simulink library "unit_testing"  (R2012b)
settings: Solver=ode45  StartTime=0.0  StopTime=10.0  RelTol=1e-3
libraries: xbsIndex_r4 x28
settings Model: Creator=ayoung  LastModifiedBy=ayoung

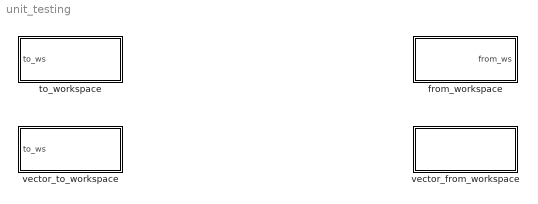
== system unit_testing ==
  from_workspace : Subsystem  mask(from_workspace){n_bits=1, bin_pt=0, arith_type=2, var_name=my_var}
      mask prompts: n_bits "Number of bits"; bin_pt "Binary point"; arith_type "Arithmetic type (ufix=0, fix=1, bool=2)"; var_name "Variable name"
      mask init:
      | blk = from_workspace_init(gcb,...
      |     'n_bits', n_bits,...
      |     'bin_pt',bin_pt,...
      |     'arith_type',arith_type,...
      |     'var_name',var_name);
      mask Display:
      | color('white');
      | text(0.5,0.5,get_param(gcb,'var_name'),'HorizontalAlignment','center');
  to_workspace : Subsystem  mask{var_name=my_var}
      mask prompts: var_name "Variable name"
      mask init:
      | var_inst = [gcb '/mvar'];
      | v = get_param(gcb,'var_name');
      | set_param(var_inst,'VariableName',v);
      mask Display:
      | color('white');
      | text(0.5,0.5,get_param(gcb,'var_name'),'HorizontalAlignment','center');
  vector_from_workspace : Subsystem  mask(vector_from_workspace){n_in=0, n_bits=0, bin_pt=0, arith_type=0, var_pfx=x}
      mask prompts: n_in "Number of inputs"; n_bits "Input width"; bin_pt "Binary point position"; arith_type "Arithmetic type (ufix=0, fix=1, bool=2)"; var_pfx "Variable name prefix"
      mask init:
      | blk = vector_from_workspace_init(gcb,...
      |     'n_in',n_in,...
      |     'n_bits',n_bits,...
      |     'bin_pt',bin_pt,...
      |     'arith_type',arith_type,...
      |     'var_pfx',var_pfx);
      mask Display:
      | color('white');
      | var_pfx = get_param(gcb,'var_pfx');
      | n_1 = 1;
      | n_N = str2num(get_param(gcb,'n_in'));
      | text(0.5,0.5,sprintf('%s_[%d..%d]',var_pfx,n_1,n_N),'HorizontalAlignment','center');
  vector_to_workspace : Subsystem  mask{n_out=8, n_bits=8, bin_pt=7, arith_type=1, var_pfx=x}
      mask prompts: n_out "Number of outputs"; n_bits "Output width"; bin_pt "Binary point position"; arith_type "Arithmetic type (ufix=0, fix=1, bool=2)"; var_pfx "Variable name prefix"
      mask init:
      | bus_inst = [gcb '/bus_expand'];
      | n_out = get_param(gcb,'n_out');
      | n_bits = get_param(gcb,'n_bits');
      | bin_pt = get_param(gcb,'bin_pt');
      | arith_type = get_param(gcb,'arith_type');
      | var_pfx = get_param(gcb,'var_pfx');
      | set_param(bus_inst,'outputNum',n_out);
      | set_param(bus_inst,'outputWidth',n_bits);
      | set_param(bus_inst,'outputBinaryPt',bin_pt);
      | set_param(bus_inst,'outputArithmeticType',arith_type);
      | set_param(bus_inst,'variablePrefix',var_pfx);
      mask Display:
      | color('white');
      | var_pfx = get_param(gcb,'var_pfx');
      | n_1 = 1;
      | n_N = str2num(get_param(gcb,'n_out'));
      | text(0.5,0.5,sprintf('%s_[%d..%d]',var_pfx,n_1,n_N),'HorizontalAlignment','center');

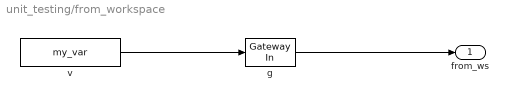
== system unit_testing/from_workspace ==
  g : xbsIndex_r4/Gateway In  gui_display_data_type=Fixed-point  arith_type=Boolean  n_bits=1  bin_pt=0  preci_type=Single  exp_width=8  frac_width=24  quantization="Round  (unbiased: +/- Inf)"  overflow=Saturate  period=1  dbl_ovrd=off  timing_constraint=None  locs_specified=off  LOCs={}  UseAsADC=off  ADCChannel='1'  inherit_from_input=off  hdl_port=on  block_type=gatewayin
  v : FromWorkspace  VariableName=my_var  SampleTime=0
  from_ws : Outport
  wires:
  v/1 -> g/1
  g/1 -> from_ws/1

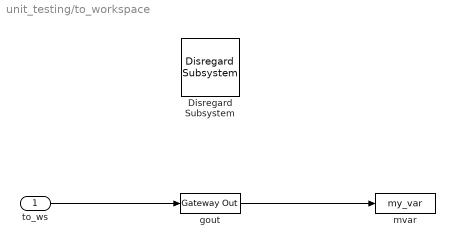
== system unit_testing/to_workspace ==
  to_ws : Inport
  Disregard Subsystem : xbsIndex_r4/Disregard Subsystem  Tag=discardX  block_type=disregard
  gout : xbsIndex_r4/Gateway Out  inherit_from_input=off  hdl_port=on  timing_constraint=None  locs_specified=off  LOCs={}  UseAsDAC=off  DACChannel='1'  block_type=gatewayout
  mvar : ToWorkspace  VariableName=my_var  SampleTime=-1  SaveFormat=Structure With Time
  wires:
  to_ws/1 -> gout/1
  gout/1 -> mvar/1

== system unit_testing/vector_from_workspace ==

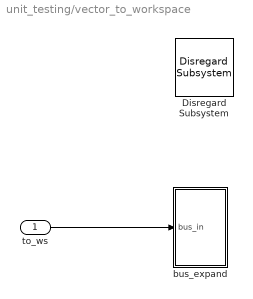
== system unit_testing/vector_to_workspace ==
  to_ws : Inport
  Disregard Subsystem : xbsIndex_r4/Disregard Subsystem  Tag=discardX  block_type=disregard
  bus_expand : Subsystem  AncestorBlock=casper_library_flow_control/bus_expand  mask(bus_expand){mode=divisions of equal size, outputNum=8, outputWidth=8, outputBinaryPt=7, outputArithmeticType=1, show_format=off, outputToWorkspace=on, variablePrefix=x, outputToModelAsWell=off}
      mask prompts: outputNum "Number of outputs:"; outputWidth "Output width:"; outputBinaryPt "Output binary point position:"; outputArithmeticType "Output arithmetic type (ufix=0, fix=1, bool=2):"; show_format "Print format string?"; outputToWorkspace "Output to workspace?"; variablePrefix "Variable name prefix:"; outputToModelAsWell "Output to model as well?"
      mask help:
      | Expands a 'bus' made using a bus_create or Xilinx
      | concat block.
      | The input will be divided into the specified number
      | of outputs with the specified arithmetic types.
      | Divisions are made from most significant bit.
      mask init:
      | bus_expand_init(gcb,...
      |     'mode', mode, ...
      |     'outputNum', outputNum, ...
      |     'outputWidth', outputWidth, ...
      |     'outputBinaryPt', outputBinaryPt, ...
      |     'outputArithmeticType', outputArithmeticType, ...
      |     'show_format', show_format, ...
      |     'outputToWorkspace', outputToWorkspace, ...
      |     'variablePrefix', variablePrefix, ...
      |     'outputToModelAsWell', outputToModelAsWell);
      settings: AttributesFormatString=8 outputs, x_?
      mask TypeOptions mode: divisions of equal size | divisions of arbitrary size
      mask Callback mode: bus_expand_callback();
      mask Callback outputWidth: bus_expand_callback();
      mask Callback outputToWorkspace: bus_expand_callback();
  wires:
  to_ws/1 -> bus_expand/1(bus_in)

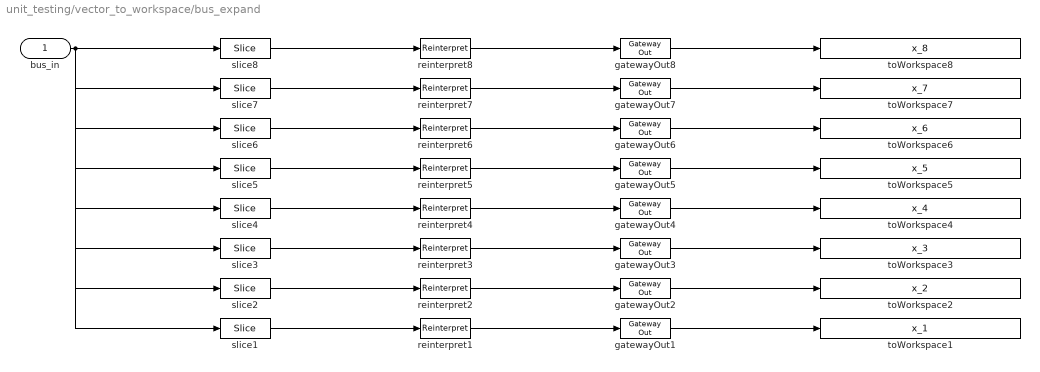
== system unit_testing/vector_to_workspace/bus_expand ==
  bus_in : Inport
  gatewayOut{1..8} (8 alike) : xbsIndex_r4/Gateway Out  inherit_from_input=off  hdl_port=off  timing_constraint=None  locs_specified=off  LOCs={}  UseAsDAC=off  DACChannel='1'  block_type=gatewayout
  reinterpret{1..8} (8 alike) : xbsIndex_r4/Reinterpret  force_arith_type=on  arith_type="Signed  (2's comp)"  force_bin_pt=on  bin_pt=7  block_type=reinterpret
  slice1 : xbsIndex_r4/Slice  nbits=8  boolean_output=off  mode=Upper Bit Location + Width  bit1=-56  base1=MSB of Input  bit0=0  base0=LSB of Input  dbl_ovrd=off  block_type=slice
  slice2 : xbsIndex_r4/Slice  nbits=8  boolean_output=off  mode=Upper Bit Location + Width  bit1=-48  base1=MSB of Input  bit0=0  base0=LSB of Input  dbl_ovrd=off  block_type=slice
  slice3 : xbsIndex_r4/Slice  nbits=8  boolean_output=off  mode=Upper Bit Location + Width  bit1=-40  base1=MSB of Input  bit0=0  base0=LSB of Input  dbl_ovrd=off  block_type=slice
  slice4 : xbsIndex_r4/Slice  nbits=8  boolean_output=off  mode=Upper Bit Location + Width  bit1=-32  base1=MSB of Input  bit0=0  base0=LSB of Input  dbl_ovrd=off  block_type=slice
  slice5 : xbsIndex_r4/Slice  nbits=8  boolean_output=off  mode=Upper Bit Location + Width  bit1=-24  base1=MSB of Input  bit0=0  base0=LSB of Input  dbl_ovrd=off  block_type=slice
  slice6 : xbsIndex_r4/Slice  nbits=8  boolean_output=off  mode=Upper Bit Location + Width  bit1=-16  base1=MSB of Input  bit0=0  base0=LSB of Input  dbl_ovrd=off  block_type=slice
  slice7 : xbsIndex_r4/Slice  nbits=8  boolean_output=off  mode=Upper Bit Location + Width  bit1=-8  base1=MSB of Input  bit0=0  base0=LSB of Input  dbl_ovrd=off  block_type=slice
  slice8 : xbsIndex_r4/Slice  nbits=8  boolean_output=off  mode=Upper Bit Location + Width  bit1=0  base1=MSB of Input  bit0=0  base0=LSB of Input  dbl_ovrd=off  block_type=slice
  toWorkspace1 : ToWorkspace  VariableName=x_1  SampleTime=-1  SaveFormat=Structure With Time
  toWorkspace2 : ToWorkspace  VariableName=x_2  SampleTime=-1  SaveFormat=Structure With Time
  toWorkspace3 : ToWorkspace  VariableName=x_3  SampleTime=-1  SaveFormat=Structure With Time
  toWorkspace4 : ToWorkspace  VariableName=x_4  SampleTime=-1  SaveFormat=Structure With Time
  toWorkspace5 : ToWorkspace  VariableName=x_5  SampleTime=-1  SaveFormat=Structure With Time
  toWorkspace6 : ToWorkspace  VariableName=x_6  SampleTime=-1  SaveFormat=Structure With Time
  toWorkspace7 : ToWorkspace  VariableName=x_7  SampleTime=-1  SaveFormat=Structure With Time
  toWorkspace8 : ToWorkspace  VariableName=x_8  SampleTime=-1  SaveFormat=Structure With Time
  wires:
  bus_in/1 -> slice8/1, slice7/1, slice6/1, slice5/1, slice4/1, slice3/1, slice2/1, slice1/1
  slice8/1 -> reinterpret8/1
  reinterpret8/1 -> gatewayOut8/1
  gatewayOut8/1 -> toWorkspace8/1
  slice7/1 -> reinterpret7/1
  reinterpret7/1 -> gatewayOut7/1
  gatewayOut7/1 -> toWorkspace7/1
  slice6/1 -> reinterpret6/1
  reinterpret6/1 -> gatewayOut6/1
  gatewayOut6/1 -> toWorkspace6/1
  slice5/1 -> reinterpret5/1
  reinterpret5/1 -> gatewayOut5/1
  gatewayOut5/1 -> toWorkspace5/1
  slice4/1 -> reinterpret4/1
  reinterpret4/1 -> gatewayOut4/1
  gatewayOut4/1 -> toWorkspace4/1
  slice3/1 -> reinterpret3/1
  reinterpret3/1 -> gatewayOut3/1
  gatewayOut3/1 -> toWorkspace3/1
  slice2/1 -> reinterpret2/1
  reinterpret2/1 -> gatewayOut2/1
  gatewayOut2/1 -> toWorkspace2/1
  slice1/1 -> reinterpret1/1
  reinterpret1/1 -> gatewayOut1/1
  gatewayOut1/1 -> toWorkspace1/1
